simulink model "HighwayLaneChangePlanner"  (R2024b)
settings: Solver=FixedStepAuto  StartTime=0.0  StopTime=10.0  RelTol=1e-3  EnableMultiTasking=on
undefined symbols (not defined in the file or in its folder): actorProfiles, Ts
(part 2 of 2)

== matlab function HighwayLaneChangePlanner/Lane Change Planner/Trajectory Optimizer/Trjaectory Optimization Block/Optimization ==
  data: planner input; EgoAndTargetStaes input; MIOGlobalStates input; MapInfo input; planner_params input; Optimizer output Bus: BusTrajectoryOptimizer; replanning input; result output
function [Optimizer, result] = optimize(planner, EgoAndTargetStaes, MIOGlobalStates, MapInfo, planner_params, replanning)

    persistent A_eq A_ineq H e1 e2 build x_prev
    
    tic; 
    Optimizer = HelperLCPlannerDefaultData.TrajectoryOptimizer;
    pp = planner_params;
    m = pp.degree;
    N = pp.num_piece;
    nvars = N * 2*(m+1);

    optimal_gap_sequence_ids = planner.optimal_gap_sequence;
    optimal_gap_sequence = planner.Gaps(optimal_gap_sequence_ids);
    EgoState = EgoAndTargetStaes.EgoFrenetState; % [s, ds, dds, l, dl, ddl]
    EgoLane = helperDetectLaneNumber(MapInfo, EgoState(4));
    MIOState = MIOGlobalStates;
    Target_gap = optimal_gap_sequence(end);
   
    %% Update Persistent Variables
    if isempty(build)
        build = true;
        [H, e1, e2] = build_matrix(planner_params);
        [A_eq, A_ineq] = build_A_matrix(build, planner_params, e1, e2);
        x_prev = zeros(nvars, 1);
    end

    if ~replanning
        x = x_prev;
        Target_MIO_State = select_target_mio(Target_gap, EgoState, MIOState, MapInfo);
        Ps = zeros(N, m+1); Pd = zeros(N, m+1);
        for i = 1:N
            base = (i-1)*2*(m+1);
            Ps(i,:) = x(base+(1:(m+1)))';
            Pd(i,:) = x(base+((m+2):(2*(m+1))))';
        end
        Optimizer.Optimal_S(1:N, 1:m+1) = Ps;
        Optimizer.Optimal_D(1:N, 1:m+1) = Pd;
        Optimizer.Target_MIO_State = Target_MIO_State;
        result = 1;
        return;
    else
        %% Setting Parameters for Optimization
        tic;
        EgoLaneCenter = MapInfo.LaneCenters(EgoLane);
        [Target_vel_min, Target_vel_max, Target_MIO_State] = select_target_vel(Target_gap, EgoState, MIOState, MapInfo, planner_params);
        bounds = struct("vs_max", pp.MaxLonVelocity, "vs_min", pp.MinLonVelocity, ...
                        "vd_max", pp.MaxLatVelocity, "vd_min", pp.MinLatVelocity, ...
                        "as_max", pp.MaxLonAccel, "as_min", -pp.MaxLonAccel, ...
                        "ad_max", pp.MaxLatAccel, "ad_min", -pp.MaxLatAccel, ...
                        "vs_terminal_min", Target_vel_min, "vs_terminal_max", Target_vel_max);
        Init_state = struct("s", 0,             "d", 0, ...
                            "vs", EgoState(2), "vd", EgoState(5), ...
                            "as", EgoState(3), "ad", EgoState(6));
    
        term_state = struct("d", Target_gap.d-(EgoState(4)-EgoLaneCenter), ...
                            "vd", 0, ...
                            "as", 0, "ad", 0);
    
        %% Optimization Implementation
    
        % 1) Equality constraints (원하는 상태 + 연속성)
        [~, beq_des]   = helperSetDesiredStateConstraints(Init_state, term_state, false, pp);
        [~, beq_cont] = helperSetContinuityConstraints(false, pp);
        b_eq = [beq_des; beq_cont];
    
        % 2) Inequality constraints (실행가능 + 안전)
        [~, b_feas] = helperSetFeasibleConstraints(e1, e2, bounds, false, pp);
        [~, b_safe] = helperSetSafetyConstraints(optimal_gap_sequence, false, pp);
        
 
        % b_ineq = b_feas;
        b_ineq = [b_feas; b_safe];
    
        % 3) 비용 (H는 생성시 고정; f=0)
        f = zeros(nvars, 1);
    
        % 4) 초기값 세팅
        % equality-only 최소노름 해 (x0가 아직 비어 있으면)
        if ~isempty(A_eq)
            % 최소노름 해: x0 = Aeq' * ((Aeq*Aeq') \ beq)
            At = A_eq.';
            M  = A_eq*At;
            % 수치 안전장치(약간의 정규화): M → M + λI
            lam = 1e-9;
            Ime = eye(size(M),'like',M);
            x0 = At * ((M + lam*Ime) \ b_eq);
        else
            x0 = zeros(nvars,1);
        end
        % 방어: NaN/Inf 제거
        bad = ~isfinite(x0);
        if any(bad), x0(bad) = 0; end
        % 길이 맞추기
        if numel(x0) < nvars
            x0(end+1:nvars) = 0;
        elseif numel(x0) > nvars
            x0 = x0(1:nvars);
        end
    
        % 4) QP 풀기
        ub = [];
        lb = [];
        opts = optimoptions('quadprog','Display','off','Algorithm','active-set', ...
                            'ConstraintTolerance',1e-8,...
                            'OptimalityTolerance',1e-8,...
                            'StepTolerance',1e-12);
        [x, ~, exitflag, output, lambda] = quadprog(H, f, A_ineq, b_ineq, A_eq, b_eq, lb, ub, x0, opts);
        fprintf('exitflag = %d\n', int32(exitflag));
        toc;
        % 5) 정규화 공간 [0, 1]에서의 Control Points로 변환
        Ps = zeros(N, m+1); Pd = zeros(N, m+1);
        for i = 1:N
            base = (i-1)*2*(m+1);
            Ps(i,:) = x(base+(1:(m+1)))';
            Pd(i,:) = x(base+((m+2):(2*(m+1))))';
        end

        % 6) Optimizer Class Update
        Optimizer.Optimal_S(1:N, 1:m+1) = Ps;
        Optimizer.Optimal_D(1:N, 1:m+1) = Pd;
        Optimizer.Target_MIO_State = Target_MIO_State;
        result = exitflag;

        % 7) Update
        x_prev = x;
    end
end
    
%% Auxilary Funtcion %%
function [H, e1, e2] = build_matrix(planner_params)
    N = planner_params.num_piece;
    m = planner_params.degree;
    dt = planner_params.PlanningResolution;

    % ====== 1) Qcore : 시간 스케일 "미적용" 저크 코어 ======
    if m < 3
        warning('degree m<3: jerk cost is identically zero. Set H=0.');
        Qcore = zeros(m+1);
    else
        % E3: (m-2) x (m+1) band matrix with [1 -3 3 -1]
        E3 = zeros(m-2, m+1);
        for r = 1:m-2
            E3(r, r:r+3) = [1 -3 3 -1];
        end
        D3    = (m*(m-1)*(m-2)) * E3;              % (m-2) x (m+1)
        G     = bernsteinGram(m-3);                % (m-2) x (m-2) SPD
        Qcore = (D3' * (G * D3));                  % no time scale here
    end

    % ====== 2) 축별 물리적 스케일을 "한 번만" 적용 ======
    % s(t) = T * p(u)  → ∫ j_s^2 dt = (1/T^3) * (Δ^3P)^T G (Δ^3P)
    % d(t) =     q(u)  → ∫ j_d^2 dt = (1/T^5) * (Δ^3P)^T G (Δ^3P)
    Qp_s = (1/dt^3) * Qcore;
    Qp_d = (1/dt^3) * Qcore;

    % 수치 안정
    Qp_s = (Qp_s + Qp_s')/2 + 1e-12*eye(m+1);
    Qp_d = (Qp_d + Qp_d')/2 + 1e-12*eye(m+1);

    % ====== 3) 전체 H (s/d 두 축 블록, N개 piece 블록대각) ======
    H_piece = blkdiag(Qp_s, Qp_d);  % 2*(m+1) x 2*(m+1)
    H   = kron(eye(N), H_piece);                  % (2N(m+1))^2

    % ====== 4) 차분 행렬 (제약에 사용) ======
    e1 = zeros(m, m+1);           % 1차 차분
    for i = 1:m,   e1(i,i) = -1; e1(i,i+1)=1; end
    e2 = zeros(m-1, m+1);         % 2차 차분
    for i = 1:m-1, e2(i,i)=1; e2(i,i+1)=-2; e2(i,i+2)=1; end
end


function G = bernsteinGram(n)
    % Gram matrix of Bernstein basis of degree n on [0,1]
    if n <= -1, G = []; return; end
    G = zeros(n+1);
    denom = (2*n + 1);
    for i = 0:n
        ci = nchoosek(n,i);
        for j = 0:n
            cj = nchoosek(n,j);
            G(i+1,j+1) = (ci*cj) / (denom * nchoosek(2*n, i+j));
        end
    end
    % 대칭화/수치안정
    G = (G + G')/2 + 1e-14*eye(n+1);
end


function [A_eq, A_ineq] = build_A_matrix(build, plannerparams, e1, e2)
    % Dummy State
    dummy_init_state = struct("s", 0, "d", 0, "vs", 0, "vd", 0, "as", 0, "ad", 0);
    dummy_term_state = struct("s", 0, "d", 0, "vs", 0, "vd", 0, "as", 0, "ad", 0);
    dummy_gap = HelperLCPlannerDefaultData.LaneChangeGap;
    dummy_bound = struct("vs_max", 0, "vs_min", 0, "vd_max", 0, "vd_min", 0, ...
                         "as_max", 0, "as_min", 0, "ad_max", 0, "ad_min", 0, ...
                         "vs_terminal_min", 0, "vs_terminal_max", 0);
    % 1) Equality constraints
    [Aeq_des, ~]   = helperSetDesiredStateConstraints(dummy_init_state, dummy_term_state, build, plannerparams);
    [Aeq_cont, ~]  = helperSetContinuityConstraints(build, plannerparams);

    % 2) Inequality constraints
    [A_feas, ~] = helperSetFeasibleConstraints(e1, e2, dummy_bound, build, plannerparams);
    [A_safe, ~] = helperSetSafetyConstraints([dummy_gap, dummy_gap, dummy_gap], build, plannerparams);

    A_eq = [Aeq_des; Aeq_cont];
    A_ineq = [A_feas; A_safe];   
    % A_ineq = A_feas;
end

function [Target_vel_low, Target_vel_high, Target_MIO_State] = select_target_vel(Target_gap, EgoState, MIOState, MapInfo, planner_params)
    NumMIOs = MIOState.NumMIOs;
    MIOStates = MIOState.MIOStates;
    LaneWidth = MapInfo.LaneWidth(1);
    feasible_coeff = planner_params.Feasible_coeff;
    maxFront = planner_params.MaxFront; 
    maxRear = planner_params.MaxRear; 
    T = planner_params.TimeHorizon;
    v_max = planner_params.MaxLonVelocity;
    a_max = planner_params.MaxLonAccel;
    ttc_max = planner_params.MaxTTC;
    Target_MIO_State = zeros(1, 6);
    % Target으로 잡아야 하는 MIO 선정
    if NumMIOs > 0
        Target_d = Target_gap.d;
        MIO_d_e = MIOStates(1:NumMIOs, 4) - (Target_d+EgoState(4));
        valid_MIO_ids = find(abs(MIO_d_e) <= LaneWidth/2);
        if ~isempty(valid_MIO_ids)
            % Valid MIO가 존재하는 경우
            valid_MIOState = MIOStates(valid_MIO_ids, :); % (n, 6)
            if size(valid_MIOState, 1) > 1
                % Valid MIO가 2대 이상인 경우, 제일 가까운 MIO로 선정
                [~, target_ids] = min(abs(valid_MIOState(:, 1) - EgoState(1)));
                target_MIOState = valid_MIOState(target_ids, :);
                MIO_pos_s = target_MIOState(1);
                MIO_vel = target_MIOState(2);
            else
                % Valid MIO가 1대인 경우
                target_MIOState = valid_MIOState(1, :);
                MIO_pos_s = target_MIOState(1);
                MIO_vel = target_MIOState(2);
            end
            Target_MIO_State(:) = target_MIOState;

            %% TTC 계산이 안되는 경우는 예외처리
            % 1. 앞 MIO가 빠른 경우
            if (MIO_pos_s - EgoState(1) - maxFront*2.0 > 0 && MIO_vel > EgoState(2))
                % 가속
                Target_vel_low = min(EgoState(2)+a_max*T*feasible_coeff, MIO_vel);
                Target_vel_low = min(Target_vel_low, v_max*feasible_coeff);
                Target_vel_high = v_max;
                return;
            end
            % 2. 뒤 MIO가 느린 경우
            if (EgoState(1) - MIO_pos_s - maxRear*2.0 > 0 && MIO_vel < EgoState(2))
                % 규정속도 내에서 가속
                Target_vel_low = min(EgoState(2)+a_max*T*feasible_coeff, v_max*feasible_coeff);
                Target_vel_high = v_max;
                return;
            end
            % 3. 앞 MIO가 느리지만, 최대 TTC 바깥인 경우
            if (MIO_pos_s - EgoState(1) - maxFront*2.0 > 0 && MIO_vel < EgoState(2))
                ttc = (MIO_pos_s - EgoState(1) - maxFront) / (EgoState(2) - MIO_vel);
                if ttc >= ttc_max
                    % 감속X
                    Target_vel_low = EgoState(2);
                    Target_vel_high = v_max;
                    return;
                end
            end
            % 4. 뒤 MIO가 빠르지만, 최대 TTC 바깥인 경우
            if (EgoState(1) - MIO_pos_s - maxRear*2.0 > 0 && MIO_vel > EgoState(2))
                ttc = (EgoState(1) - MIO_pos_s - maxRear) / (MIO_vel - EgoState(2));
                if ttc >= ttc_max
                    % 가속
                    Target_vel_low = min(EgoState(2)+a_max*T*feasible_coeff, MIO_vel);
                    Target_vel_low = min(Target_vel_low, v_max*feasible_coeff);
                    Target_vel_high = v_max;
                    return;
                end
            end

            %% 나머지 경우 Target Velocity Generation Algorithms
            %   - Parameters : s_0, v_0, T, a_acc, a_brk, s_M(T)
            %   - Unknown : [v_min(T), v_max(T)]
            [Target_vel_low, Target_vel_high] = helperCalculateTargetstates(EgoState, MIO_pos_s, MIO_vel, ...
                                                                            planner_params, feasible_coeff);
        else
            % Valid MIO가 없는 경우, 규정속도 내에서 가속
            Target_vel_low = min(EgoState(2)+a_max*T*feasible_coeff, v_max*feasible_coeff);
            Target_vel_high = v_max;
        end
    else
        % MIO 자체가 잡히지 않는 경우, 규정속도 내에서 가속
        Target_vel_low = min(EgoState(2)+a_max*T*feasible_coeff, v_max*feasible_coeff);
        Target_vel_high = v_max;
    end
end


function Target_MIO_State = select_target_mio(Target_gap, EgoState, MIOState, MapInfo)
    NumMIOs = MIOState.NumMIOs;
    MIOStates = MIOState.MIOStates;
    LaneWidth = MapInfo.LaneWidth(1);
    Target_MIO_State = zeros(1, 6);
    % Target으로 잡아야 하는 MIO 선정
    if NumMIOs > 0
        Target_d = Target_gap.d;
        MIO_d_e = MIOStates(1:NumMIOs, 4) - (Target_d+EgoState(4));
        valid_MIO_ids = find(abs(MIO_d_e) <= LaneWidth/2);
        if ~isempty(valid_MIO_ids)
            % Valid MIO가 존재하는 경우
            valid_MIOState = MIOStates(valid_MIO_ids, :); % (n, 6)
            if size(valid_MIOState, 1) > 1
                % Valid MIO가 2대 이상인 경우, 제일 가까운 MIO로 선정
                [~, target_ids] = min(abs(valid_MIOState(:, 1) - EgoState(1)));
                target_MIOState = valid_MIOState(target_ids, :);
            else
                % Valid MIO가 1대인 경우
                target_MIOState = valid_MIOState(1, :);
            end
            Target_MIO_State(:) = target_MIOState;
        end 
    end
end

== matlab function HighwayLaneChangePlanner/Lane Change Planner/Trajectory Optimizer/Event Trigger (Decision) ==
  data: signal output; Optimal_gap_sequence input; Gaps input; Target_Lane input
function signal = Trigger(Optimal_gap_sequence, Gaps, Target_Lane)
    signal = false;
    target_gap_id = Optimal_gap_sequence(end);
    target_gap = Gaps(target_gap_id);
    
    if ~(Target_Lane == 0)
        prev_global_lane_idx = Target_Lane;
        if target_gap.global_lane_idx ~= prev_global_lane_idx
            signal = true;
            fprintf("current_target : %d\n", int32(target_gap.global_lane_idx));
            fprintf("prev_target : %d\n", int32(prev_global_lane_idx));
        end
    end
    signal = false;
end

== matlab function HighwayLaneChangePlanner/Lane Change Planner/Spatio Temporal Safety Region/Frenet State Converter Global & Relative ==
  data: EgoAndTargetStates output Bus: BusEgoAndTargetStates; Ego input; TargetActorsWorld input; MapInfo input; EgoAndTargetRelativeStates output Bus: BusEgoAndTargetRelativeStates; Actors input; ego_lane output
function [EgoAndTargetStates, EgoAndTargetRelativeStates, ego_lane] = frenetStateConverter(Ego,... 
                                                                                 TargetActorsWorld,...
                                                                                 MapInfo, Actors)
                                                   
coder.inline('never');
persistent RefPathFrenet

% Load all actor's path points
refPath = MapInfo.GlobalPlanPoints(1:MapInfo.NumGlobalPlanPoints,:);


if isempty(RefPathFrenet)
    % Initialization : GlobalWaypoints
    RefPathFrenet = referencePathFrenet(refPath);   
else
    % Check for a change in the reference path
    if ~isequal(RefPathFrenet.Waypoints, refPath) 
        refPathNew = referencePathFrenet(refPath);
        RefPathFrenet.Waypoints = refPathNew.Waypoints;
    end
end

% Initialize output bus
egoAndTargetStates = HelperLCPlannerDefaultData.EgoAndTargetStates;
egoAndTargetRelativeStates = HelperLCPlannerDefaultData.EgoAndTargetRelativeStates;


kapa = deg2rad(Ego.AngularVelocity(3))/norm(Ego.Velocity);
if (isnan(kapa) || isinf(kapa))
    kapa = 0;
end
egoState = [Ego.Position(1:2), deg2rad(Ego.Yaw), kapa, norm(Ego.Velocity(1:2),2), norm(Ego.Acceleration(1:2), 2)];% Update the acceleration state

% Frenet States : [x, y, theta, kappa, velocity, acceleration]
% global2frenet : internal function
egoFrenetState = global2frenet(RefPathFrenet, egoState);
numTargets = TargetActorsWorld.NumActors;
targetStates = zeros(numTargets, 6);
targetFrenetStates = zeros(numTargets, 6);
targetIDs = zeros(numTargets,1);

targetRelativeStates = zeros(numTargets, 6);
targetRelativeFrenetStates = zeros(numTargets, 6);

for i=1:numTargets
    vel = norm(TargetActorsWorld.Actors(i).Velocity(1:2));
    kappa = deg2rad(TargetActorsWorld.Actors(i).AngularVelocity(3))/vel;
    if (isnan(kappa) || isinf(kappa))
        kappa = 0;
    end

    targetStates(i,:) = [TargetActorsWorld.Actors(i).Position(1:2),...
                       deg2rad(TargetActorsWorld.Actors(i).Yaw), kappa,...
                       vel, 0];

    targetIDs(i,1) = TargetActorsWorld.Actors(i).ActorID;
    targetFrenetStates(i,:) = global2frenet(RefPathFrenet, targetStates(i,:));

    targetRelativeStates(i, :) = targetStates(i, :) - egoState;

    targetRelativeFrenetStates(i, 1) = targetFrenetStates(i, 1) - egoFrenetState(1); % s
    targetRelativeFrenetStates(i, 2) = targetFrenetStates(i, 2) - egoFrenetState(2); % ds
    targetRelativeFrenetStates(i, 3) = targetFrenetStates(i, 3) - egoFrenetState(3); % dds
    targetRelativeFrenetStates(i, 4) = targetFrenetStates(i, 4) - egoFrenetState(4); % l
    targetRelativeFrenetStates(i, 5) = targetFrenetStates(i, 5) - egoFrenetState(5); % dl
    targetRelativeFrenetStates(i, 6) = targetFrenetStates(i, 6) - egoFrenetState(6); % ddl 


    % Update the lateral and logitudinal  frenet states to zero when the
    % speed is zero.
    if abs(targetStates(i,5)) < 1e-3
        targetFrenetStates(i,2) = 0;
        targetFrenetStates(i,5) = 0;

    end
end

egoAndTargetStates.NumTargetActors = numTargets;
egoAndTargetStates.TargetGlobalStates(1:numTargets,:) = targetStates;
egoAndTargetStates.TargetFrenetStates(1:numTargets,:) = targetFrenetStates;
egoAndTargetStates.TargetIDs(1:numTargets,:) = targetIDs;
egoAndTargetStates.EgoGlobalState = egoState;
egoAndTargetStates.EgoFrenetState = egoFrenetState;
EgoAndTargetStates = egoAndTargetStates;

egoAndTargetRelativeStates.NumTargetActors = numTargets;
egoAndTargetRelativeStates.TargetRelativeStates(1:numTargets,:) = targetRelativeStates;
egoAndTargetRelativeStates.TargetRelativeFrenetStates(1:numTargets,:) = targetRelativeFrenetStates;
egoAndTargetRelativeStates.TargetIDs(1:numTargets,:) = targetIDs;
egoAndTargetRelativeStates.EgoGlobalFrenetState = egoFrenetState;
EgoAndTargetRelativeStates = egoAndTargetRelativeStates;


%%%%%%%%%%%%%%%% Ego 차량 차선 결정 %%%%%%%%%%%%%%%%%%

ego_length = Actors(1).Length;
ego_width = Actors(1).Width;
ego_frenet = [egoFrenetState(1); egoFrenetState(4)];
ego_frenet_yaw = rad2deg(atan2(egoFrenetState(5), egoFrenetState(2)));
if abs(ego_frenet_yaw) < 1e-5
    ego_frenet_yaw = 0;
end
rotationMatrix = [cosd(ego_frenet_yaw), -sind(ego_frenet_yaw); sind(ego_frenet_yaw), cosd(ego_frenet_yaw)];

if ego_frenet_yaw > 0
    ego_front_right = rotationMatrix * [ego_length/2; -ego_width/2] + ego_frenet;
    ego_lane = helperDetectLaneNumber(MapInfo, ego_front_right(2));
elseif ego_frenet_yaw < 0
    ego_front_left = rotationMatrix * [ego_length/2; ego_width/2] + ego_frenet;
    ego_lane = helperDetectLaneNumber(MapInfo, ego_front_left(2));
else
    ego_lane = helperDetectLaneNumber(MapInfo, egoFrenetState(4));
end

end
